simulink model "frame_differencing_vehicle_detection"  (R2015b)
settings: Solver=VariableStepAuto  StartTime=0.0  StopTime=inf  RelTol=1e-3
undefined symbols (not defined in the file): gray, Rec, SDTV, strel
libraries: visiontextngfix x5, visionsinks x3, visionstatistics x2, visionconversions x2, dspvision x1, visionmorphops x1, simulink x1
settings Model: Creator=Monty  LastModifiedBy=Monty

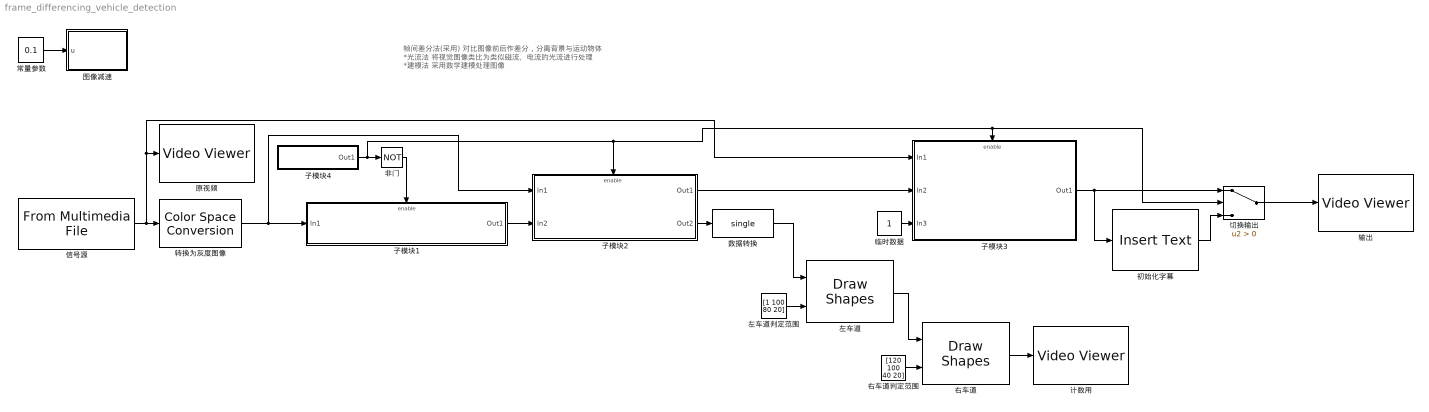
== system frame_differencing_vehicle_detection ==
  note: 帧间差分法(采用)
      | 对比图像前后作差分，分离背景与运动物体
      | *光流法
      | 将视觉图像类比为类似磁流、电流的光流进行处理
      | *建模法
      | 采用数学建模处理图像
  临时数据 : Constant  OutDataTypeStr=int16
  信号源 : dspvision/From Multimedia File  inputFilename=E:\STUDY\CIRCUIT\Matlab 2015b win64\Matlab 2015b win64\MATLAB\R2015b\toolbox\vision\visiondata\viptraffic.avi  loop=on  numPlays=inf  outputStreams=Video only  videoDataType=single  audioDataType=int16  inheritSampleTime=on  userDefinedSampleTime=1/30  noAudioOutput=off  isIntensityVideo=off  fourcc=RGB  colorVideoFormat=One multidimensional signal  outputEOF=off  dataOrg=Column-major  audioFrameSize=1024  computeAudioFrameSize=off  outSamplingMode=Sample based
  切换输出 : Switch  Criteria=u2 > Threshold
  初始化字幕 : visiontextngfix/Insert Text  inputType=Obsolete  theText='Initialing'  getTextLocFrom=Specify via dialog  textLoc=[50 50]  getTextColorFrom=Specify via dialog  textColor=[1 1 1]  getTextIntensityFrom=Specify via dialog  textIntensity=0  getTextOpacityFrom=Specify via dialog  textOpacity=1.0  dummyVar2=0  dummyVar3=0  dummyVar4=0  imagePorts=One multidimensional signal  isInputTransposed=off  fontFace=LucidaSansRegular  dummyVar1=0  blockFontSize=14  antiAliased=on
  原视频 : visionsinks/Video Viewer  inputType=Obsolete7b  imagePorts=One multidimensional signal  useColorMap=off  colormapValue=gray(256)  specRange=off  minInputVal=0  maxInputVal=255  FigPos=[701 310 409.6 167.2]  AxisZoom=on  trueSizedOnce=off  OpenAtMdlStart=on  DefaultConfigurationName=vipscopes.VideoViewerScopeCfg
  右车道 : visiontextngfix/Draw Shapes  shape=Rectangles  fill=on  lineWidth=2  fillClrSource=Specify via dialog  display=White  intensity=200  color=[200 255 100]  opacity=0.6  viewport=Entire image  antialiasing=off  inType=Obsolete  imagePorts=One multidimensional signal  prodOutputMode=Binary point scaling  prodOutputWordLength=32  prodOutputFracLength=14  memoryMode=Specify word length  memoryWordLength=16  memoryFracLength=14  roundingMode=Floor  overflowMode=off
  右车道判定范围 : Constant  Value=[120 100 40 20]
  图像减速 : MATLAB Function  TreatAsAtomicUnit=on
  子模块1 : Subsystem
      mask Display:
      | disp('提取背景\n邱剑楠')
      | port_label('input',1,'原始视频输入口')
      | port_label('output',1,'背景图像')
  子模块2 : Subsystem
      mask Display:
      | disp('识别车辆\n邱剑楠')
      | port_label('input',1,'原始视频输入口')
      | port_label('input',2,'背景图像')
      | port_label('output',1,'位置')
      | port_label('output',2,'Blob图像')
  子模块3 : Subsystem
      mask Display:
      | disp('显示单元\n邱剑楠')
      | port_label('input',1,'原始视频输入口')
      | port_label('input',2,'位置信息')
      | port_label('input',3,'计数')
      | port_label('output',1,'结果输出')
  子模块4 : Subsystem
      mask Display:
      | disp('控制信号\n邱剑楠')
      | port_label('output',1,'')
  左车道 : visiontextngfix/Draw Shapes  shape=Rectangles  fill=on  lineWidth=2  fillClrSource=Specify via dialog  display=White  intensity=200  color=[200 255 100]  opacity=0.6  viewport=Entire image  antialiasing=off  inType=Obsolete  imagePorts=One multidimensional signal  prodOutputMode=Binary point scaling  prodOutputWordLength=32  prodOutputFracLength=14  memoryMode=Specify word length  memoryWordLength=16  memoryFracLength=14  roundingMode=Floor  overflowMode=off
  左车道判定范围 : Constant  Value=[1 100 80 20]
  常量参数 : Constant  Value=0.1
  数据转换 : DataTypeConversion  OutDataTypeStr=single
  计数用 : visionsinks/Video Viewer  inputType=Obsolete7b  imagePorts=One multidimensional signal  useColorMap=off  colormapValue=gray(256)  specRange=off  minInputVal=0  maxInputVal=255  FigPos=[1115.4 308.4 409.6 167.2]  AxisZoom=on  trueSizedOnce=off  OpenAtMdlStart=on  DefaultConfigurationName=vipscopes.VideoViewerScopeCfg
  转换为灰度图像 : visionconversions/Color Space  Conversion  conversion=Obsolete  conversionActive=R'G'B' to intensity  wp_str=D65  rec=Rec. 601 (SDTV)  sys=1125/60/2:1  imagePorts=One multidimensional signal
  输出 : visionsinks/Video Viewer  inputType=Obsolete7b  imagePorts=One multidimensional signal  useColorMap=off  colormapValue=gray(256)  specRange=off  minInputVal=0  maxInputVal=255  FigPos=[269 308.4 409.6 167.2]  AxisZoom=on  trueSizedOnce=off  OpenAtMdlStart=on  DefaultConfigurationName=vipscopes.VideoViewerScopeCfg
  非门 : Logic  Operator=NOT  AllPortsSameDT=off  OutDataTypeStr=boolean
  wires:
  常量参数/1 -> 图像减速/1(u)
  信号源/1 -> 子模块3/1(In1), 原视频/1, 转换为灰度图像/1
  子模块1/1(Out1) -> 子模块2/2(In2)
  子模块2/1(Out1) -> 子模块3/2(In2)
  子模块4/1(Out1) -> 子模块3/Enable, 切换输出/2, 子模块2/Enable, 非门/1
  非门/1 -> 子模块1/Enable
  转换为灰度图像/1 -> 子模块2/1(In1), 子模块1/1(In1)
  子模块3/1(Out1) -> 初始化字幕/1, 切换输出/1
  切换输出/1 -> 输出/1
  初始化字幕/1 -> 切换输出/3
  临时数据/1 -> 子模块3/3(In3)
  子模块2/2(Out2) -> 数据转换/1
  数据转换/1 -> 左车道/1
  左车道判定范围/1 -> 左车道/2
  左车道/1 -> 右车道/1
  右车道判定范围/1 -> 右车道/2
  右车道/1 -> 计数用/1

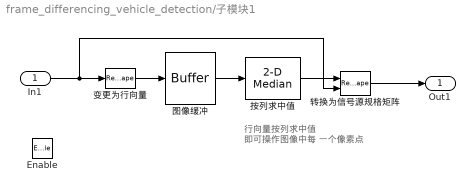
== system frame_differencing_vehicle_detection/子模块1 ==
  note: 行向量按列求中值
      | 即可操作图像中每
      | 一个像素点
  In1 : Inport
  Enable : EnablePort
  变更为行向量 : Reshape  OutputDimensionality=Row vector (2-D)
  图像缓冲 : Buffer  N=40  V=5  TreatMby1Signals=One channel  OutputFrames=off
  按列求中值 : visionstatistics/2-D Median  sortAlg=Quick sort  directionMode=Each column  dimension=1  treatSBRowAsCol=on  outputDataTypeStr=Inherit: Same as accumulator  outputLastDataTypeStr=Inherit: Same as accumulator  outputMin=[]  outputMax=[]  accumMode=Binary point scaling  accumWordLength=32  accumFracLength=0  accumDataTypeStr=fixdt([],32,0)  accumLastDataTypeStr=fixdt([],32,0)  roundingMode=Floor  overflowMode=off
      settings: allowOverrides=off
  转换为信号源规格矩阵 : Reshape  OutputDimensionality=Derive from reference input port
  Out1 : Outport
  wires:
  图像缓冲/1 -> 按列求中值/1
  按列求中值/1 -> 转换为信号源规格矩阵/1
  转换为信号源规格矩阵/1 -> Out1/1
  In1/1 -> 转换为信号源规格矩阵/2, 变更为行向量/1
  变更为行向量/1 -> 图像缓冲/1

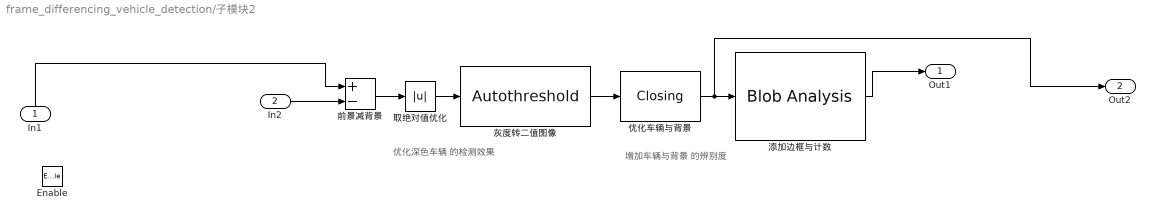
== system frame_differencing_vehicle_detection/子模块2 ==
  note: 增加车辆与背景
      | 的辨别度
  note: 优化深色车辆
      | 的检测效果
  In1 : Inport
  In2 : Inport  Port=2
  Enable : EnablePort
  优化车辆与背景 : visionmorphops/Closing  nhoodsrc=Specify via dialog  strel=strel('square',7)
  前景减背景 : Sum  Inputs=+-
  取绝对值优化 : Abs
  添加边框与计数 : visionstatistics/Blob Analysis  Tag=vipblks_row_conv  area=off  centroid=off  bBox=on  majorAxis=off  minorAxis=off  angle=off  eccentricity=off  equivDiameterSq=off  extent=off  perimeter=off  maxBlobs=10  warnIfNumBlobsExceeded=on  isCount=off  useMinArea=on  minArea=350  useMaxArea=on  maxArea=4000  excludeBorderBlob=off  outDT=double  isOutVarDim=off  isFill=on  fillValues=-1  conn=8  isLabel=off  outputMode=Binary point scaling  outputWordLength=32  outputFracLength=16  firstCoeffMode=Binary point scaling  firstCoeffWordLength=16  firstCoeffFracLength=14  secondCoeffMode=Binary point scaling  secondCoeffWordLength=32  secondCoeffFracLength=16  accumMode=Binary point scaling  accumWordLength=32  accumFracLength=0  prodOutputMode=Binary point scaling  prodOutputWordLength=32  prodOutputFracLength=16  roundingMode=Floor  overflowMode=off
  灰度转二值图像 : visionconversions/Autothreshold  operator=>  threshOut=off  effMetricOut=off  userDefinedRange=off  umin=0  umax=255  outOfRngOpt=Warn and saturate  scaleThreshold=off  scaleFactor=1  P1Mode=Specify word length  P1WordLength=32  P1FracLength=30  P2Mode=Specify word length  P2WordLength=32  P2FracLength=22  P3Mode=Specify word length  P3WordLength=32  P3FracLength=14  P4Mode=Binary point scaling  P4WordLength=32  P4FracLength=15  Q1Mode=Specify word length  Q1WordLength=32  Q1FracLength=16  EMMode=Specify word length  EMWordLength=16  EMFracLength=14  roundingMode=Floor  overflowMode=off
  Out1 : Outport
  Out2 : Outport  Port=2
  wires:
  添加边框与计数/1 -> Out1/1
  取绝对值优化/1 -> 灰度转二值图像/1
  In1/1 -> 前景减背景/1
  灰度转二值图像/1 -> 优化车辆与背景/1
  优化车辆与背景/1 -> Out2/1, 添加边框与计数/1
  In2/1 -> 前景减背景/2
  前景减背景/1 -> 取绝对值优化/1

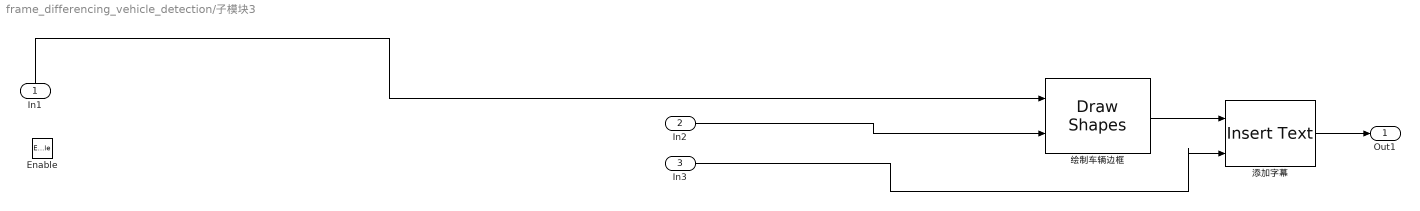
== system frame_differencing_vehicle_detection/子模块3 ==
  In1 : Inport
  In2 : Inport  Port=2
  In3 : Inport  Port=3
  Enable : EnablePort
  添加字幕 : visiontextngfix/Insert Text  inputType=Obsolete  theText='%3d car are found'  getTextLocFrom=Specify via dialog  textLoc=[10 6]  getTextColorFrom=Specify via dialog  textColor=[1 1 1]  getTextIntensityFrom=Specify via dialog  textIntensity=0  getTextOpacityFrom=Specify via dialog  textOpacity=1.0  dummyVar2=0  dummyVar3=0  dummyVar4=0  imagePorts=One multidimensional signal  isInputTransposed=off  fontFace=LucidaSansRegular  dummyVar1=0  blockFontSize=14  antiAliased=on
  绘制车辆边框 : visiontextngfix/Draw Shapes  shape=Rectangles  fill=off  lineWidth=2  fillClrSource=Specify via dialog  display=User-specified value  intensity=200  color=[0 0 1]  opacity=0.6  viewport=Entire image  antialiasing=off  inType=Obsolete  imagePorts=One multidimensional signal  prodOutputMode=Binary point scaling  prodOutputWordLength=32  prodOutputFracLength=14  memoryMode=Specify word length  memoryWordLength=16  memoryFracLength=15  roundingMode=Floor  overflowMode=off
  Out1 : Outport
  wires:
  添加字幕/1 -> Out1/1
  In2/1 -> 绘制车辆边框/2
  In3/1 -> 添加字幕/2
  绘制车辆边框/1 -> 添加字幕/1
  In1/1 -> 绘制车辆边框/1

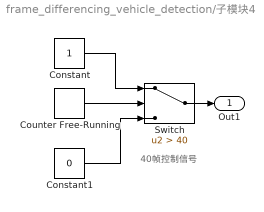
== system frame_differencing_vehicle_detection/子模块4 ==
  note: 40帧控制信号
  Constant : Constant
  Constant1 : Constant  Value=0
  Counter Free-Running : simulink/Sources/Counter Free-Running  NumBits=16  tsamp=1/15
  Switch : Switch  Criteria=u2 > Threshold  Threshold=40
  Out1 : Outport
  wires:
  Constant/1 -> Switch/1
  Counter Free-Running/1 -> Switch/2
  Constant1/1 -> Switch/3
  Switch/1 -> Out1/1

== matlab function frame_differencing_vehicle_detection/图像减速 ==
  data: u input
function fcn(u)
%#codegen

pause(u);
